simulink model "lab7"  (R2022b)
settings: Solver=VariableStepAuto  StartTime=0.0  StopTime=10.0  RelTol=1e-3
undefined symbols (not defined in the file): k1, k2, L1, L2, S1, S2, T1, T2, T3
settings Model: Creator=dambi  LastModifiedBy=dambi

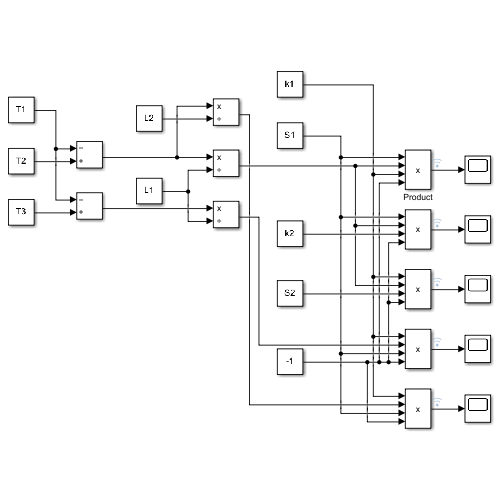
[thumbnail: Simulink's stored preview of the top-level diagram]
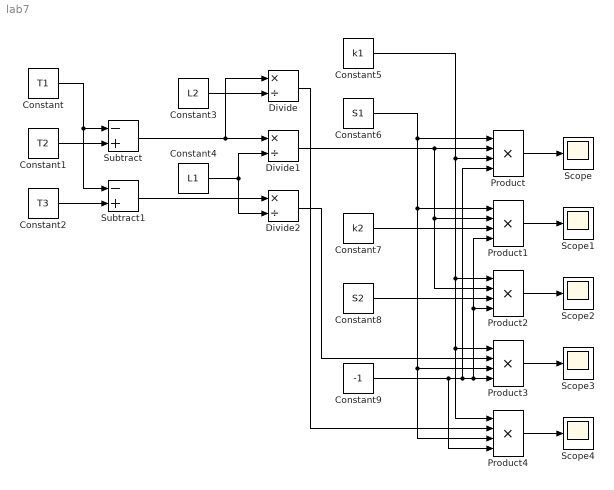
== system lab7 ==
  Constant : Constant  Value=T1
  Constant1 : Constant  Value=T2
  Constant2 : Constant  Value=T3
  Constant3 : Constant  Value=L2
  Constant4 : Constant  Value=L1
  Constant5 : Constant  Value=k1
  Constant6 : Constant  Value=S1
  Constant7 : Constant  Value=k2
  Constant8 : Constant  Value=S2
  Constant9 : Constant  Value=-1
  Divide : Product  Inputs=*/
  Divide1 : Product  Inputs=*/
  Divide2 : Product  Inputs=*/
  Product{,1..4} (5 alike) : Product  Inputs=4
  Scope{,1..4} (5 alike) : Scope
  Subtract : Sum  Inputs=-+
  Subtract1 : Sum  Inputs=-+
  wires:
  Subtract1/1 -> Divide2/1
  Subtract/1 -> Divide/1, Divide1/1
  Constant3/1 -> Divide/2
  Constant4/1 -> Divide2/2, Divide1/2
  Constant6/1 -> Product/1, Product1/1, Product3/3, Product4/3
  Constant5/1 -> Product/3, Product2/1, Product3/1, Product4/1
  Product4/1 -> Scope4/1
  Product/1 -> Scope/1
  Product1/1 -> Scope1/1
  Product2/1 -> Scope2/1
  Product3/1 -> Scope3/1
  Constant7/1 -> Product1/3
  Constant8/1 -> Product2/3
  Constant9/1 -> Product4/4, Product/4, Product2/4, Product1/4, Product3/4
  Divide/1 -> Product4/2
  Divide1/1 -> Product1/2, Product2/2, Product/2
  Divide2/1 -> Product3/2
  Constant/1 -> Subtract1/1, Subtract/1
  Constant2/1 -> Subtract1/2
  Constant1/1 -> Subtract/2
